simulink model "GPI_Test1_Ball_Beam"  (R2018b)
settings: Solver=ode14x  StartTime=0.0  StopTime=10.0  FixedStep=0.0001  RelTol=1e-3
values from neighbouring files (symbols this model uses):
  k = -m*g*d/L/(J/R^2+m)    (= -4.53935338144e-06)    [Parameter.m]
  k0 = sys.Denominator{1}(9)    [Parameter.m]
  k1 = sys.Denominator{1}(8)    [Parameter.m]
  k2 = sys.Denominator{1}(7)    [Parameter.m]
  k3 = sys.Denominator{1}(6)    [Parameter.m]
  k4 = sys.Denominator{1}(5)    [Parameter.m]
  k5 = sys.Denominator{1}(4)    [Parameter.m]
  k6 = sys.Denominator{1}(3)    [Parameter.m]
  k7 = sys.Denominator{1}(2)    [Parameter.m]
  wt = 20    [Parameter.m]
  Xit = 1    [Parameter.m]
settings Model: Creator=cheng  LastModifiedBy=cheng

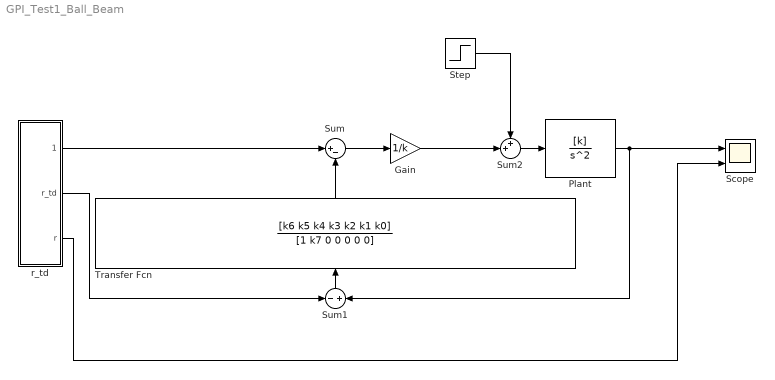
== system GPI_Test1_Ball_Beam ==
  Gain : Gain  Gain=1/k
  Plant : TransferFcn  Numerator=[k]  Denominator=[1 0 0]
  Scope : Scope  NumInputPorts=2
  Step : Step  Time=5  After=1000  SampleTime=0
  Sum : Sum  Inputs=|+-
  Sum1 : Sum  Inputs=-|+
  Sum2 : Sum  Inputs=++|
  Transfer Fcn : TransferFcn  Numerator=[k6 k5 k4 k3 k2 k1 k0]  Denominator=[1 k7 0 0 0 0 0]
  r_td : Subsystem
  wires:
  Plant/1 -> Sum1/2, Scope/1
  Gain/1 -> Sum2/2
  Sum/1 -> Gain/1
  Transfer Fcn/1 -> Sum/2
  Sum1/1 -> Transfer Fcn/1
  r_td/2(r_td) -> Sum1/1
  r_td/1(rdd_td) -> Sum/1
  Sum2/1 -> Plant/1
  Step/1 -> Sum2/1
  r_td/3(r) -> Scope/2

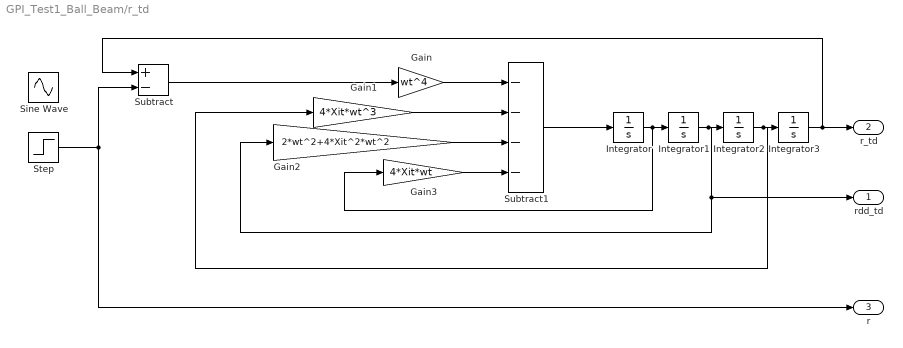
== system GPI_Test1_Ball_Beam/r_td ==
  Gain : Gain  Gain=wt^4
  Gain1 : Gain  Gain=4*Xit*wt^3
  Gain2 : Gain  Gain=2*wt^2+4*Xit^2*wt^2
  Gain3 : Gain  Gain=4*Xit*wt
  Integrator{,1..3} (4 alike) : Integrator
  Sine Wave : Sin  SampleTime=0
  Step : Step  SampleTime=0
  Subtract : Sum  Inputs=+-
  Subtract1 : Sum  Inputs=----
  rdd_td : Outport
  r_td : Outport  Port=2
  r : Outport  Port=3
  wires:
  Step/1 -> Subtract/2, r/1
  Integrator1/1 -> Gain2/1, rdd_td/1, Integrator2/1
  Integrator3/1 -> Subtract/1, r_td/1
  Integrator2/1 -> Gain1/1, Integrator3/1
  Integrator/1 -> Gain3/1, Integrator1/1
  Subtract/1 -> Gain/1
  Gain/1 -> Subtract1/1
  Gain1/1 -> Subtract1/2
  Gain2/1 -> Subtract1/3
  Gain3/1 -> Subtract1/4
  Subtract1/1 -> Integrator/1
